simulink model "chap04_CA1"  (R2021a)
settings: Solver=FixedStepDiscrete  StartTime=0.0  StopTime=30  FixedStep=0.001  RelTol=1e-3
undefined symbols (not defined in the file): DiscIntNeverNeededParam
libraries: simulink x4
(part 2 of 4)

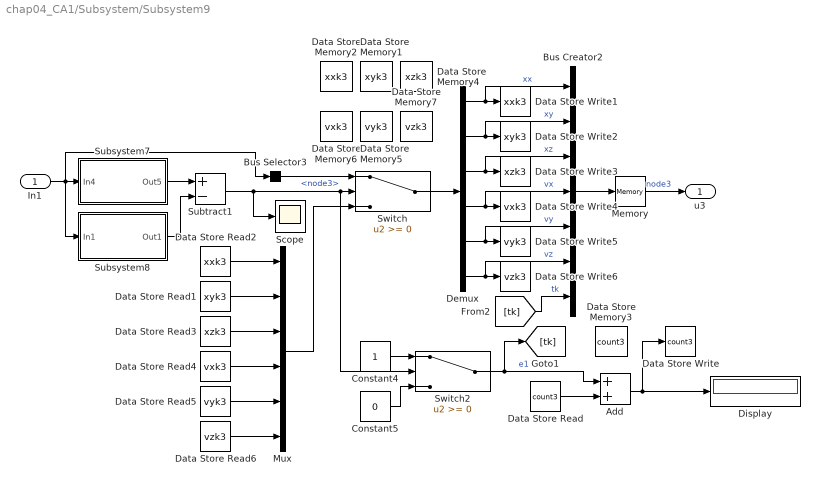
== system chap04_CA1/Subsystem/Subsystem9 ==
  In1 : Inport
  Add : Sum
  Bus Creator2 : BusCreator  Inputs=7
  Bus Selector3 : BusSelector  OutputSignals=state(t).node3
  Constant4 : Constant
  Constant5 : Constant  Value=0
  Data Store Memory1 : DataStoreMemory  DataStoreName=xyk3  ReadBeforeWriteMsg=warning  WriteAfterWriteMsg=warning  WriteAfterReadMsg=warning  ShowAdditionalParam=off
  Data Store Memory2 : DataStoreMemory  DataStoreName=xxk3  ReadBeforeWriteMsg=warning  WriteAfterWriteMsg=warning  WriteAfterReadMsg=warning  ShowAdditionalParam=off
  Data Store Memory3 : DataStoreMemory  DataStoreName=count3  ReadBeforeWriteMsg=warning  WriteAfterWriteMsg=warning  WriteAfterReadMsg=warning  ShowAdditionalParam=off
  Data Store Memory4 : DataStoreMemory  DataStoreName=xzk3  ReadBeforeWriteMsg=warning  WriteAfterWriteMsg=warning  WriteAfterReadMsg=warning  ShowAdditionalParam=off
  Data Store Memory5 : DataStoreMemory  DataStoreName=vyk3  ReadBeforeWriteMsg=warning  WriteAfterWriteMsg=warning  WriteAfterReadMsg=warning  ShowAdditionalParam=off
  Data Store Memory6 : DataStoreMemory  DataStoreName=vxk3  ReadBeforeWriteMsg=warning  WriteAfterWriteMsg=warning  WriteAfterReadMsg=warning  ShowAdditionalParam=off
  Data Store Memory7 : DataStoreMemory  DataStoreName=vzk3  ReadBeforeWriteMsg=warning  WriteAfterWriteMsg=warning  WriteAfterReadMsg=warning  ShowAdditionalParam=off
  Data Store Read : DataStoreRead  DataStoreName=count3  IndexOptions=Index vector (dialog)  Indices=1  OutputSizes=1
  Data Store Read1 : DataStoreRead  DataStoreName=xyk3  IndexOptions=Index vector (dialog)  Indices=1  OutputSizes=1
  Data Store Read2 : DataStoreRead  DataStoreName=xxk3  IndexOptions=Index vector (dialog)  Indices=1  OutputSizes=1
  Data Store Read3 : DataStoreRead  DataStoreName=xzk3  IndexOptions=Index vector (dialog)  Indices=1  OutputSizes=1
  Data Store Read4 : DataStoreRead  DataStoreName=vxk3  IndexOptions=Index vector (dialog)  Indices=1  OutputSizes=1
  Data Store Read5 : DataStoreRead  DataStoreName=vyk3  IndexOptions=Index vector (dialog)  Indices=1  OutputSizes=1
  Data Store Read6 : DataStoreRead  DataStoreName=vzk3  IndexOptions=Index vector (dialog)  Indices=1  OutputSizes=1
  Data Store Write : DataStoreWrite  DataStoreName=count3  IndexOptions=Index vector (dialog)  Indices=1  OutputSizes=1
  Data Store Write1 : DataStoreWrite  DataStoreName=xxk3  IndexOptions=Index vector (dialog)  Indices=1  OutputSizes=1
  Data Store Write2 : DataStoreWrite  DataStoreName=xyk3  IndexOptions=Index vector (dialog)  Indices=1  OutputSizes=1
  Data Store Write3 : DataStoreWrite  DataStoreName=xzk3  IndexOptions=Index vector (dialog)  Indices=1  OutputSizes=1
  Data Store Write4 : DataStoreWrite  DataStoreName=vxk3  IndexOptions=Index vector (dialog)  Indices=1  OutputSizes=1
  Data Store Write5 : DataStoreWrite  DataStoreName=vyk3  IndexOptions=Index vector (dialog)  Indices=1  OutputSizes=1
  Data Store Write6 : DataStoreWrite  DataStoreName=vzk3  IndexOptions=Index vector (dialog)  Indices=1  OutputSizes=1
  Demux : Demux  Outputs=6
  Display : Display
  Memory : Memory
  Mux : Mux  Inputs=6
  Scope : Scope
  Subsystem7 : Subsystem
  Subsystem8 : Subsystem
  Subtract1 : Sum  Inputs=+-
  Switch : Switch
  Switch2 : Switch
  u3 : Outport
  wires:
  Data Store Read6/1 -> Mux/6
  Switch/1 -> Demux/1
  Demux/2 -> Bus Creator2/2, Data Store Write2/1  "xy"
  Bus Selector3/1 -> Switch/1  "<node3>"
  Demux/1 -> Bus Creator2/1, Data Store Write1/1  "xx"
  Switch2/1 -> [tk], Add/1  "e1"
  Demux/6 -> Bus Creator2/6, Data Store Write6/1  "vz"
  Demux/3 -> Bus Creator2/3, Data Store Write3/1  "xz"
  Data Store Read2/1 -> Mux/1
  Constant4/1 -> Switch2/1
  Mux/1 -> Switch/3
  Data Store Read3/1 -> Mux/3
  Add/1 -> Data Store Write/1, Display/1
  Demux/4 -> Bus Creator2/4, Data Store Write4/1  "vx"
  Memory/1 -> u3/1  "node3"
  Data Store Read5/1 -> Mux/5
  Data Store Read4/1 -> Mux/4
  Data Store Read1/1 -> Mux/2
  Constant5/1 -> Switch2/3
  Demux/5 -> Bus Creator2/5, Data Store Write5/1  "vy"
  Data Store Read/1 -> Add/2
  Bus Creator2/1 -> Memory/1
  Subtract1/1 -> Scope/1, Switch/2, Switch2/2
  [tk] -> Bus Creator2/7  "tk"
  Subsystem8/1(Out1) -> Subtract1/2
  In1/1 -> Bus Selector3/1, Subsystem7/1(In4), Subsystem8/1(In1)
  Subsystem7/1(Out5) -> Subtract1/1

== system chap04_CA1/Subsystem2/Subsystem ==
  dx : Inport
  dy : Inport  Port=2
  dz : Inport  Port=3
  ut1x : Inport  Port=4
  ut1y : Inport  Port=5
  ut1z : Inport  Port=6
  Add : Sum
  Add1 : Sum
  Add2 : Sum
  Add3 : Sum  Inputs=-+
  Add4 : Sum  Inputs=-+
  Add5 : Sum  Inputs=-+
  Bus Creator1 : BusCreator  Inputs=6
  Constant : Constant  Value=-1
  Constant1 : Constant
  Constant2 : Constant  Value=0
  Discrete-Time Integrator{,15..17} (4 alike) : DiscreteIntegrator  SampleTime=-1  ICPrevOutput=DiscIntNeverNeededParam  ICPrevScaledInput=DiscIntNeverNeededParam
  Discrete-Time Integrator14 : DiscreteIntegrator  InitialCondition=-1  SampleTime=-1  ICPrevOutput=DiscIntNeverNeededParam  ICPrevScaledInput=DiscIntNeverNeededParam
  Discrete-Time Integrator5 : DiscreteIntegrator  InitialCondition=1  SampleTime=-1  ICPrevOutput=DiscIntNeverNeededParam  ICPrevScaledInput=DiscIntNeverNeededParam
  node1 : Outport
  wires:
  ut1y/1 -> Add1/2
  ut1z/1 -> Add2/2
  Discrete-Time Integrator17/1 -> Discrete-Time Integrator15/1, Bus Creator1/5  "vy"
  Discrete-Time Integrator/1 -> Discrete-Time Integrator5/1, Bus Creator1/6  "vz"
  ut1x/1 -> Add/2
  Discrete-Time Integrator16/1 -> Bus Creator1/4, Discrete-Time Integrator14/1  "vx"
  Bus Creator1/1 -> node1/1  "node1"
  Add5/1 -> Bus Creator1/3  "xz"
  Add4/1 -> Bus Creator1/2  "xy"
  Add3/1 -> Bus Creator1/1  "xx"
  Add/1 -> Discrete-Time Integrator16/1
  Add1/1 -> Discrete-Time Integrator17/1
  Add2/1 -> Discrete-Time Integrator/1
  dy/1 -> Add1/1
  dz/1 -> Add2/1
  dx/1 -> Add/1
  Discrete-Time Integrator14/1 -> Add3/2
  Discrete-Time Integrator5/1 -> Add5/2
  Discrete-Time Integrator15/1 -> Add4/2
  Constant/1 -> Add3/1
  Constant1/1 -> Add4/1
  Constant2/1 -> Add5/1

== system chap04_CA1/Subsystem2/Subsystem1 ==
  dx : Inport
  dy : Inport  Port=2
  dz : Inport  Port=3
  ut2x : Inport  Port=4
  ut2y : Inport  Port=5
  ut2z : Inport  Port=6
  Add : Sum
  Add1 : Sum
  Add2 : Sum
  Add3 : Sum  Inputs=-+
  Add4 : Sum  Inputs=-+
  Add5 : Sum  Inputs=-+
  Bus Creator1 : BusCreator  Inputs=6
  Constant : Constant
  Constant1 : Constant
  Constant2 : Constant  Value=0
  Discrete-Time Integrator : DiscreteIntegrator  SampleTime=-1  ICPrevOutput=DiscIntNeverNeededParam  ICPrevScaledInput=DiscIntNeverNeededParam
  Discrete-Time Integrator14 : DiscreteIntegrator  InitialCondition=1.5  SampleTime=-1  ICPrevOutput=DiscIntNeverNeededParam  ICPrevScaledInput=DiscIntNeverNeededParam
  Discrete-Time Integrator15 : DiscreteIntegrator  InitialCondition=0.5  SampleTime=-1  ICPrevOutput=DiscIntNeverNeededParam  ICPrevScaledInput=DiscIntNeverNeededParam
  Discrete-Time Integrator16 : DiscreteIntegrator  SampleTime=-1  ICPrevOutput=DiscIntNeverNeededParam  ICPrevScaledInput=DiscIntNeverNeededParam
  Discrete-Time Integrator17 : DiscreteIntegrator  SampleTime=-1  ICPrevOutput=DiscIntNeverNeededParam  ICPrevScaledInput=DiscIntNeverNeededParam
  Discrete-Time Integrator5 : DiscreteIntegrator  InitialCondition=1  SampleTime=-1  ICPrevOutput=DiscIntNeverNeededParam  ICPrevScaledInput=DiscIntNeverNeededParam
  node2 : Outport
  wires:
  Bus Creator1/1 -> node2/1  "node2"
  Discrete-Time Integrator16/1 -> Bus Creator1/4, Discrete-Time Integrator14/1  "vx"
  Discrete-Time Integrator/1 -> Discrete-Time Integrator5/1, Bus Creator1/6  "vz"
  Discrete-Time Integrator17/1 -> Bus Creator1/5, Discrete-Time Integrator15/1  "vy"
  dx/1 -> Add/1
  dy/1 -> Add1/1
  dz/1 -> Add2/1
  Add2/1 -> Discrete-Time Integrator/1
  Add1/1 -> Discrete-Time Integrator17/1
  Add/1 -> Discrete-Time Integrator16/1
  ut2x/1 -> Add/2
  ut2y/1 -> Add1/2
  ut2z/1 -> Add2/2
  Constant2/1 -> Add5/1
  Constant1/1 -> Add4/1
  Discrete-Time Integrator14/1 -> Add3/2
  Discrete-Time Integrator15/1 -> Add4/2
  Discrete-Time Integrator5/1 -> Add5/2
  Constant/1 -> Add3/1
  Add3/1 -> Bus Creator1/1  "xx"
  Add4/1 -> Bus Creator1/2  "xy"
  Add5/1 -> Bus Creator1/3  "xz"

== system chap04_CA1/Subsystem2/Subsystem2 ==
  dx : Inport
  dy : Inport  Port=2
  dz : Inport  Port=3
  ut3x : Inport  Port=4
  ut3y : Inport  Port=5
  ut3z : Inport  Port=6
  Add : Sum
  Add1 : Sum
  Add2 : Sum
  Add3 : Sum  Inputs=-+
  Add4 : Sum  Inputs=-+
  Add5 : Sum  Inputs=-+
  Bus Creator1 : BusCreator  Inputs=6
  Constant : Constant  Value=-2
  Constant1 : Constant  Value=0
  Constant2 : Constant  Value=0
  Discrete-Time Integrator : DiscreteIntegrator  SampleTime=-1  ICPrevOutput=DiscIntNeverNeededParam  ICPrevScaledInput=DiscIntNeverNeededParam
  Discrete-Time Integrator14 : DiscreteIntegrator  InitialCondition=-1  SampleTime=-1  ICPrevOutput=DiscIntNeverNeededParam  ICPrevScaledInput=DiscIntNeverNeededParam
  Discrete-Time Integrator15 : DiscreteIntegrator  InitialCondition=-1  SampleTime=-1  ICPrevOutput=DiscIntNeverNeededParam  ICPrevScaledInput=DiscIntNeverNeededParam
  Discrete-Time Integrator16 : DiscreteIntegrator  SampleTime=-1  ICPrevOutput=DiscIntNeverNeededParam  ICPrevScaledInput=DiscIntNeverNeededParam
  Discrete-Time Integrator17 : DiscreteIntegrator  SampleTime=-1  ICPrevOutput=DiscIntNeverNeededParam  ICPrevScaledInput=DiscIntNeverNeededParam
  Discrete-Time Integrator5 : DiscreteIntegrator  InitialCondition=0.5  SampleTime=-1  ICPrevOutput=DiscIntNeverNeededParam  ICPrevScaledInput=DiscIntNeverNeededParam
  node3 : Outport
  wires:
  Discrete-Time Integrator17/1 -> Discrete-Time Integrator15/1, Bus Creator1/5  "vy"
  Discrete-Time Integrator/1 -> Discrete-Time Integrator5/1, Bus Creator1/6  "vz"
  Discrete-Time Integrator16/1 -> Bus Creator1/4, Discrete-Time Integrator14/1  "vx"
  Bus Creator1/1 -> node3/1  "node3"
  ut3x/1 -> Add/2
  ut3y/1 -> Add1/2
  Add/1 -> Discrete-Time Integrator16/1
  dy/1 -> Add1/1
  Add1/1 -> Discrete-Time Integrator17/1
  Add2/1 -> Discrete-Time Integrator/1
  dz/1 -> Add2/1
  dx/1 -> Add/1
  ut3z/1 -> Add2/2
  Constant2/1 -> Add5/1
  Constant1/1 -> Add4/1
  Discrete-Time Integrator14/1 -> Add3/2
  Discrete-Time Integrator15/1 -> Add4/2
  Discrete-Time Integrator5/1 -> Add5/2
  Constant/1 -> Add3/1
  Add3/1 -> Bus Creator1/1  "xx"
  Add4/1 -> Bus Creator1/2  "xy"
  Add5/1 -> Bus Creator1/3  "xz"

== system chap04_CA1/Subsystem2/Subsystem3 ==
  dx : Inport
  dy : Inport  Port=2
  dz : Inport  Port=3
  ut4x : Inport  Port=4
  ut4y : Inport  Port=5
  ut4z : Inport  Port=6
  Add : Sum
  Add1 : Sum
  Add2 : Sum
  Add3 : Sum  Inputs=-+
  Add4 : Sum  Inputs=-+
  Add5 : Sum  Inputs=-+
  Bus Creator1 : BusCreator  Inputs=6
  Constant : Constant  Value=2
  Constant1 : Constant  Value=0
  Constant2 : Constant  Value=0
  Discrete-Time Integrator : DiscreteIntegrator  SampleTime=-1  ICPrevOutput=DiscIntNeverNeededParam  ICPrevScaledInput=DiscIntNeverNeededParam
  Discrete-Time Integrator14 : DiscreteIntegrator  InitialCondition=4  SampleTime=-1  ICPrevOutput=DiscIntNeverNeededParam  ICPrevScaledInput=DiscIntNeverNeededParam
  Discrete-Time Integrator15 : DiscreteIntegrator  InitialCondition=-1  SampleTime=-1  ICPrevOutput=DiscIntNeverNeededParam  ICPrevScaledInput=DiscIntNeverNeededParam
  Discrete-Time Integrator16 : DiscreteIntegrator  SampleTime=-1  ICPrevOutput=DiscIntNeverNeededParam  ICPrevScaledInput=DiscIntNeverNeededParam
  Discrete-Time Integrator17 : DiscreteIntegrator  SampleTime=-1  ICPrevOutput=DiscIntNeverNeededParam  ICPrevScaledInput=DiscIntNeverNeededParam
  Discrete-Time Integrator5 : DiscreteIntegrator  InitialCondition=0.5  SampleTime=-1  ICPrevOutput=DiscIntNeverNeededParam  ICPrevScaledInput=DiscIntNeverNeededParam
  node4 : Outport
  wires:
  Bus Creator1/1 -> node4/1  "node4"
  Discrete-Time Integrator16/1 -> Discrete-Time Integrator14/1, Bus Creator1/4  "vx"
  Discrete-Time Integrator/1 -> Discrete-Time Integrator5/1, Bus Creator1/6  "vz"
  Discrete-Time Integrator17/1 -> Bus Creator1/5, Discrete-Time Integrator15/1  "vy"
  ut4x/1 -> Add/2
  ut4y/1 -> Add1/2
  Add/1 -> Discrete-Time Integrator16/1
  dy/1 -> Add1/1
  Add1/1 -> Discrete-Time Integrator17/1
  Add2/1 -> Discrete-Time Integrator/1
  dz/1 -> Add2/1
  dx/1 -> Add/1
  ut4z/1 -> Add2/2
  Constant2/1 -> Add5/1
  Constant1/1 -> Add4/1
  Discrete-Time Integrator14/1 -> Add3/2
  Discrete-Time Integrator15/1 -> Add4/2
  Discrete-Time Integrator5/1 -> Add5/2
  Constant/1 -> Add3/1
  Add3/1 -> Bus Creator1/1  "xx"
  Add4/1 -> Bus Creator1/2  "xy"
  Add5/1 -> Bus Creator1/3  "xz"

== system chap04_CA1/Subsystem2/Subsystem4 ==
  dx : Inport
  dy : Inport  Port=2
  dz : Inport  Port=3
  ut5x : Inport  Port=4
  ut5y : Inport  Port=5
  ut5z : Inport  Port=6
  Add : Sum
  Add1 : Sum
  Add2 : Sum
  Add3 : Sum  Inputs=-+
  Add4 : Sum  Inputs=-+
  Add5 : Sum  Inputs=-+
  Bus Creator1 : BusCreator  Inputs=6
  Constant : Constant  Value=-1
  Constant1 : Constant  Value=-1
  Constant2 : Constant  Value=0
  Discrete-Time Integrator{,5,16..17} (4 alike) : DiscreteIntegrator  SampleTime=-1  ICPrevOutput=DiscIntNeverNeededParam  ICPrevScaledInput=DiscIntNeverNeededParam
  Discrete-Time Integrator14 : DiscreteIntegrator  InitialCondition=0.7  SampleTime=-1  ICPrevOutput=DiscIntNeverNeededParam  ICPrevScaledInput=DiscIntNeverNeededParam
  Discrete-Time Integrator15 : DiscreteIntegrator  InitialCondition=-1.7  SampleTime=-1  ICPrevOutput=DiscIntNeverNeededParam  ICPrevScaledInput=DiscIntNeverNeededParam
  node5 : Outport
  wires:
  Discrete-Time Integrator17/1 -> Discrete-Time Integrator15/1, Bus Creator1/5  "vy"
  Discrete-Time Integrator/1 -> Discrete-Time Integrator5/1, Bus Creator1/6  "vz"
  Discrete-Time Integrator16/1 -> Bus Creator1/4, Discrete-Time Integrator14/1  "vx"
  Bus Creator1/1 -> node5/1  "node5"
  ut5x/1 -> Add/2
  ut5y/1 -> Add1/2
  Add/1 -> Discrete-Time Integrator16/1
  dy/1 -> Add1/1
  Add1/1 -> Discrete-Time Integrator17/1
  Add2/1 -> Discrete-Time Integrator/1
  dz/1 -> Add2/1
  dx/1 -> Add/1
  ut5z/1 -> Add2/2
  Constant2/1 -> Add5/1
  Constant1/1 -> Add4/1
  Discrete-Time Integrator14/1 -> Add3/2
  Discrete-Time Integrator15/1 -> Add4/2
  Discrete-Time Integrator5/1 -> Add5/2
  Constant/1 -> Add3/1
  Add3/1 -> Bus Creator1/1  "xx"
  Add4/1 -> Bus Creator1/2  "xy"
  Add5/1 -> Bus Creator1/3  "xz"

== system chap04_CA1/Subsystem2/Subsystem5 ==
  dx : Inport
  dy : Inport  Port=2
  dz : Inport  Port=3
  ut6x : Inport  Port=4
  ut6y : Inport  Port=5
  ut6z : Inport  Port=6
  Add : Sum
  Add1 : Sum
  Add2 : Sum
  Add3 : Sum  Inputs=-+
  Add4 : Sum  Inputs=-+
  Add5 : Sum  Inputs=-+
  Bus Creator1 : BusCreator  Inputs=6
  Constant : Constant
  Constant1 : Constant  Value=-1
  Constant2 : Constant  Value=0
  Discrete-Time Integrator{,5,16..17} (4 alike) : DiscreteIntegrator  SampleTime=-1  ICPrevOutput=DiscIntNeverNeededParam  ICPrevScaledInput=DiscIntNeverNeededParam
  Discrete-Time Integrator14 : DiscreteIntegrator  InitialCondition=3  SampleTime=-1  ICPrevOutput=DiscIntNeverNeededParam  ICPrevScaledInput=DiscIntNeverNeededParam
  Discrete-Time Integrator15 : DiscreteIntegrator  InitialCondition=-1.5  SampleTime=-1  ICPrevOutput=DiscIntNeverNeededParam  ICPrevScaledInput=DiscIntNeverNeededParam
  node6 : Outport
  wires:
  Bus Creator1/1 -> node6/1  "node6"
  Discrete-Time Integrator16/1 -> Discrete-Time Integrator14/1, Bus Creator1/4  "vx"
  Discrete-Time Integrator/1 -> Discrete-Time Integrator5/1, Bus Creator1/6  "vz"
  Discrete-Time Integrator17/1 -> Bus Creator1/5, Discrete-Time Integrator15/1  "vy"
  ut6x/1 -> Add/2
  ut6y/1 -> Add1/2
  Add/1 -> Discrete-Time Integrator16/1
  dy/1 -> Add1/1
  Add1/1 -> Discrete-Time Integrator17/1
  Add2/1 -> Discrete-Time Integrator/1
  dz/1 -> Add2/1
  dx/1 -> Add/1
  ut6z/1 -> Add2/2
  Constant2/1 -> Add5/1
  Constant1/1 -> Add4/1
  Discrete-Time Integrator14/1 -> Add3/2
  Discrete-Time Integrator15/1 -> Add4/2
  Discrete-Time Integrator5/1 -> Add5/2
  Constant/1 -> Add3/1
  Add3/1 -> Bus Creator1/1  "xx"
  Add4/1 -> Bus Creator1/2  "xy"
  Add5/1 -> Bus Creator1/3  "xz"

== system chap04_CA1/Subsystem2/Subsystem6 ==
  Clock1 : Clock
  Constant1 : Constant  Value=0.25
  Constant3 : Constant  Value=0.25
  Constant9 : Constant  Value=0.1
  Discrete Derivative : simulink/Discrete/Discrete Derivative  gainval=1.0  ICPrevScaledInput=1000  OutMin=[]  OutMax=[]  OutDataType=fixdt(1, 16)  OutScaling=2^-10  DoSatur=off
  Discrete Derivative1 : simulink/Discrete/Discrete Derivative  gainval=1.0  ICPrevScaledInput=-0.25  OutMin=[]  OutMax=[]  OutDataType=fixdt(1, 16)  OutScaling=2^-10  DoSatur=off
  Discrete Derivative2 : simulink/Discrete/Discrete Derivative  gainval=1.0  ICPrevScaledInput=249.9  OutMin=[]  OutMax=[]  OutDataType=fixdt(1, 16)  OutScaling=2^-10  DoSatur=off
  Product{,1..3} (4 alike) : Product
  Sum : Sum  Inputs=|++
  Trigonometric Function2 : Trigonometry
  Trigonometric Function3 : Trigonometry  Operator=cos
  r : Constant
  xx : Outport
  xy : Outport  Port=2
  xz : Outport  Port=3
  vx : Outport  Port=4
  vy : Outport  Port=5
  vz : Outport  Port=6
  wires:
  Discrete Derivative/1 -> vx/1
  Discrete Derivative1/1 -> vy/1
  Sum/1 -> Discrete Derivative2/1, xz/1
  Discrete Derivative2/1 -> vz/1
  Product/1 -> xx/1, Discrete Derivative/1
  Product1/1 -> xy/1, Discrete Derivative1/1
  Product2/1 -> Trigonometric Function2/1, Trigonometric Function3/1
  Trigonometric Function3/1 -> Product/1
  Constant9/1 -> Product3/2
  Clock1/1 -> Product3/1, Product2/2
  Trigonometric Function2/1 -> Product1/2
  Constant3/1 -> Product2/1
  r/1 -> Product/2, Product1/1
  Product3/1 -> Sum/1
  Constant1/1 -> Sum/2

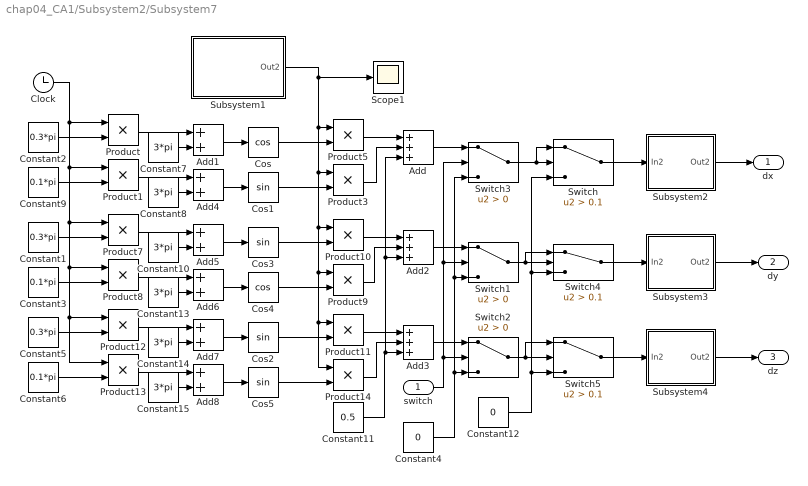
== system chap04_CA1/Subsystem2/Subsystem7 ==
  switch : Inport
  Add : Sum  Inputs=+++
  Add{1,4..8} (6 alike) : Sum
  Add2 : Sum  Inputs=+++
  Add3 : Sum  Inputs=+++
  Clock : Clock
  Constant1 : Constant  Value=0.3*pi
  Constant{7..8,10,13..15} (6 alike) : Constant  Value=3*pi
  Constant11 : Constant  Value=0.5
  Constant12 : Constant  Value=0
  Constant2 : Constant  Value=0.3*pi
  Constant3 : Constant  Value=0.1*pi
  Constant4 : Constant  Value=0
  Constant5 : Constant  Value=0.3*pi
  Constant6 : Constant  Value=0.1*pi
  Constant9 : Constant  Value=0.1*pi
  Cos : Trigonometry  Operator=cos
  Cos{1..3,5} (4 alike) : Trigonometry
  Cos4 : Trigonometry  Operator=cos
  Product{,1,3,5,7..14} (12 alike) : Product
  Scope1 : Scope
  Subsystem1 : Subsystem
  Subsystem2 : Subsystem
  Subsystem3 : Subsystem
  Subsystem4 : Subsystem
  Switch : Switch  Criteria=u2 > Threshold  Threshold=0.1
  Switch1 : Switch  Criteria=u2 > Threshold
  Switch2 : Switch  Criteria=u2 > Threshold
  Switch3 : Switch  Criteria=u2 > Threshold
  Switch4 : Switch  Criteria=u2 > Threshold  Threshold=0.1
  Switch5 : Switch  Criteria=u2 > Threshold  Threshold=0.1
  dx : Outport
  dy : Outport  Port=2
  dz : Outport  Port=3
  wires:
  Add/1 -> Switch3/1
  Add2/1 -> Switch1/1
  Switch2/1 -> Switch5/1, Switch5/2
  Product11/1 -> Add3/1
  Constant6/1 -> Product13/2
  Subsystem1/1(Out2) -> Scope1/1, Product11/1, Product14/1, Product9/1, Product10/1, Product3/1, Product5/1
  Product14/1 -> Add3/2
  Cos2/1 -> Product11/2
  Cos5/1 -> Product14/2
  Constant5/1 -> Product12/2
  Product12/1 -> Add7/1
  Product13/1 -> Add8/1
  Clock/1 -> Product/1, Product13/1, Product12/1, Product8/1, Product7/1, Product1/1
  Product10/1 -> Add2/1
  Product8/1 -> Add6/1
  Product7/1 -> Add5/1
  Constant1/1 -> Product7/2
  Cos4/1 -> Product9/2
  Cos3/1 -> Product10/2
  Product9/1 -> Add2/2
  Constant3/1 -> Product8/2
  Constant9/1 -> Product1/2
  Product3/1 -> Add/2
  Cos/1 -> Product5/2
  Add3/1 -> Switch2/1
  Cos1/1 -> Product3/2
  switch/1 -> Switch2/2, Switch1/2, Switch3/2
  Constant4/1 -> Switch3/3, Switch1/3, Switch2/3
  Product5/1 -> Add/1
  Constant2/1 -> Product/2
  Product/1 -> Add1/1
  Product1/1 -> Add4/1
  Switch1/1 -> Switch4/1, Switch4/2
  Switch3/1 -> Switch/1, Switch/2
  Switch/1 -> Subsystem2/1(In2)
  Constant12/1 -> Switch/3, Switch4/3, Switch5/3
  Constant11/1 -> Add/3, Add2/3, Add3/3
  Switch4/1 -> Subsystem3/1(In2)
  Switch5/1 -> Subsystem4/1(In2)
  Subsystem2/1(Out2) -> dx/1
  Subsystem3/1(Out2) -> dy/1
  Subsystem4/1(Out2) -> dz/1
  Add1/1 -> Cos/1
  Constant7/1 -> Add1/2
  Add4/1 -> Cos1/1
  Constant8/1 -> Add4/2
  Add5/1 -> Cos3/1
  Constant10/1 -> Add5/2
  Add6/1 -> Cos4/1
  Constant13/1 -> Add6/2
  Add7/1 -> Cos2/1
  Constant14/1 -> Add7/2
  Add8/1 -> Cos5/1
  Constant15/1 -> Add8/2

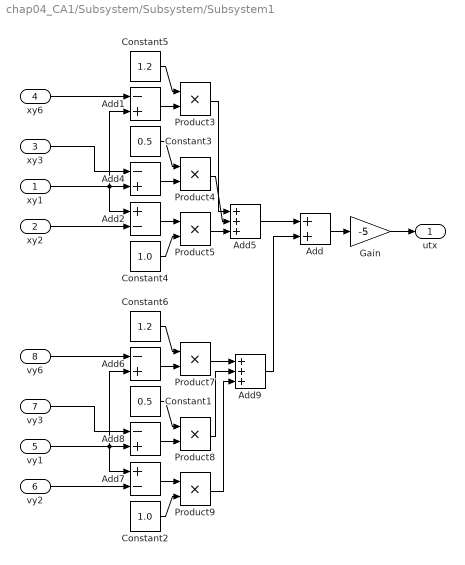
== system chap04_CA1/Subsystem/Subsystem/Subsystem1 ==
  xy1 : Inport
  xy2 : Inport  Port=2
  xy3 : Inport  Port=3
  xy6 : Inport  Port=4
  vy1 : Inport  Port=5
  vy2 : Inport  Port=6
  vy3 : Inport  Port=7
  vy6 : Inport  Port=8
  Add : Sum
  Add{1,4,6,8} (4 alike) : Sum  Inputs=-+
  Add2 : Sum  Inputs=+-
  Add5 : Sum  Inputs=+++
  Add7 : Sum  Inputs=+-
  Add9 : Sum  Inputs=+++
  Constant1 : Constant  Value=0.5
  Constant2 : Constant  Value=1.0
  Constant3 : Constant  Value=0.5
  Constant4 : Constant  Value=1.0
  Constant5 : Constant  Value=1.2
  Constant6 : Constant  Value=1.2
  Gain : Gain  Gain=-5
  Product{3..5,7..9} (6 alike) : Product
  utx : Outport
  wires:
  Product8/1 -> Add9/2
  Product9/1 -> Add9/3
  Constant1/1 -> Product8/1
  Add8/1 -> Product8/2
  vy1/1 -> Add6/2, Add8/2, Add7/1
  Constant2/1 -> Product9/2
  Add7/1 -> Product9/1
  vy3/1 -> Add8/1
  vy2/1 -> Add7/2
  vy6/1 -> Add6/1
  Constant6/1 -> Product7/1
  Add6/1 -> Product7/2
  Product7/1 -> Add9/1
  Product3/1 -> Add5/1
  Add1/1 -> Product3/2
  Constant5/1 -> Product3/1
  xy6/1 -> Add1/1
  xy2/1 -> Add2/2
  xy3/1 -> Add4/1
  Add2/1 -> Product5/1
  Constant4/1 -> Product5/2
  xy1/1 -> Add2/1, Add4/2, Add1/2
  Add4/1 -> Product4/2
  Constant3/1 -> Product4/1
  Product5/1 -> Add5/3
  Product4/1 -> Add5/2
  Add5/1 -> Add/1
  Add/1 -> Gain/1
  Gain/1 -> utx/1
  Add9/1 -> Add/2

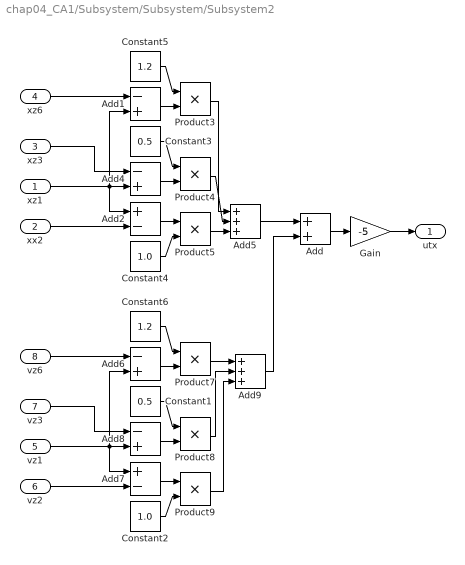
== system chap04_CA1/Subsystem/Subsystem/Subsystem2 ==
  xz1 : Inport
  xx2 : Inport  Port=2
  xz3 : Inport  Port=3
  xz6 : Inport  Port=4
  vz1 : Inport  Port=5
  vz2 : Inport  Port=6
  vz3 : Inport  Port=7
  vz6 : Inport  Port=8
  Add : Sum
  Add{1,4,6,8} (4 alike) : Sum  Inputs=-+
  Add2 : Sum  Inputs=+-
  Add5 : Sum  Inputs=+++
  Add7 : Sum  Inputs=+-
  Add9 : Sum  Inputs=+++
  Constant1 : Constant  Value=0.5
  Constant2 : Constant  Value=1.0
  Constant3 : Constant  Value=0.5
  Constant4 : Constant  Value=1.0
  Constant5 : Constant  Value=1.2
  Constant6 : Constant  Value=1.2
  Gain : Gain  Gain=-5
  Product{3..5,7..9} (6 alike) : Product
  utx : Outport
  wires:
  Product4/1 -> Add5/2
  Product5/1 -> Add5/3
  Constant3/1 -> Product4/1
  Add4/1 -> Product4/2
  xz1/1 -> Add1/2, Add4/2, Add2/1
  Constant4/1 -> Product5/2
  Add2/1 -> Product5/1
  xz3/1 -> Add4/1
  xx2/1 -> Add2/2
  xz6/1 -> Add1/1
  Constant5/1 -> Product3/1
  Add1/1 -> Product3/2
  Product3/1 -> Add5/1
  Product7/1 -> Add9/1
  Add6/1 -> Product7/2
  Constant6/1 -> Product7/1
  vz6/1 -> Add6/1
  vz2/1 -> Add7/2
  vz3/1 -> Add8/1
  Add7/1 -> Product9/1
  Constant2/1 -> Product9/2
  vz1/1 -> Add7/1, Add8/2, Add6/2
  Add8/1 -> Product8/2
  Constant1/1 -> Product8/1
  Product9/1 -> Add9/3
  Product8/1 -> Add9/2
  Add5/1 -> Add/1
  Add/1 -> Gain/1
  Gain/1 -> utx/1
  Add9/1 -> Add/2

== system chap04_CA1/Subsystem/Subsystem/Subsystem6 ==
  xx1 : Inport
  xx2 : Inport  Port=2
  xx3 : Inport  Port=3
  xx6 : Inport  Port=4
  vx1 : Inport  Port=5
  vx2 : Inport  Port=6
  vx3 : Inport  Port=7
  vx6 : Inport  Port=8
  Add : Sum
  Add{1,4,6,8} (4 alike) : Sum  Inputs=-+
  Add2 : Sum  Inputs=+-
  Add5 : Sum  Inputs=+++
  Add7 : Sum  Inputs=+-
  Add9 : Sum  Inputs=+++
  Constant1 : Constant  Value=0.5
  Constant2 : Constant  Value=1.0
  Constant3 : Constant  Value=0.5
  Constant4 : Constant  Value=1.0
  Constant5 : Constant  Value=1.2
  Constant6 : Constant  Value=1.2
  Gain : Gain  Gain=-5
  Product{3..5,7..9} (6 alike) : Product
  utx : Outport
  wires:
  Product4/1 -> Add5/2
  Product5/1 -> Add5/3
  Constant3/1 -> Product4/1
  Add4/1 -> Product4/2
  xx1/1 -> Add1/2, Add4/2, Add2/1
  Constant4/1 -> Product5/2
  Add5/1 -> Add/1
  Add9/1 -> Add/2
  Add2/1 -> Product5/1
  xx3/1 -> Add4/1
  xx2/1 -> Add2/2
  xx6/1 -> Add1/1
  Constant5/1 -> Product3/1
  Add1/1 -> Product3/2
  Product3/1 -> Add5/1
  Product7/1 -> Add9/1
  Add6/1 -> Product7/2
  Constant6/1 -> Product7/1
  vx6/1 -> Add6/1
  vx2/1 -> Add7/2
  vx3/1 -> Add8/1
  Add7/1 -> Product9/1
  Constant2/1 -> Product9/2
  vx1/1 -> Add7/1, Add8/2, Add6/2
  Add8/1 -> Product8/2
  Constant1/1 -> Product8/1
  Product9/1 -> Add9/3
  Product8/1 -> Add9/2
  Add/1 -> Gain/1
  Gain/1 -> utx/1

== system chap04_CA1/Subsystem/Subsystem1/Subsystem1 ==
  xy5 : Inport
  xy0 : Inport  Port=2
  xy3 : Inport  Port=3
  xy4 : Inport  Port=4
  vy5 : Inport  Port=5
  vy0 : Inport  Port=6
  vy3 : Inport  Port=7
  vy4 : Inport  Port=8
  Add : Sum
  Add1 : Sum  Inputs=-+
  Add10 : Sum  Inputs=-+
  Add2 : Sum  Inputs=+-
  Add4 : Sum  Inputs=-+
  Add5 : Sum  Inputs=+++
  Add6 : Sum  Inputs=+-
  Add8 : Sum  Inputs=+++
  Add9 : Sum  Inputs=+-
  Constant3 : Constant  Value=1.2
  Constant4 : Constant  Value=1.5
  Constant5 : Constant  Value=1.2
  Constant6 : Constant  Value=1.5
  Constant7 : Constant  Value=2.0
  Constant8 : Constant  Value=2.0
  Gain : Gain  Gain=-5.0
  Product{3..5,7..9} (6 alike) : Product
  uty : Outport
  wires:
  vy0/1 -> Add6/2
  Constant8/1 -> Product7/2
  Add6/1 -> Product7/1
  Product7/1 -> Add8/3
  Product3/1 -> Add5/1
  xy0/1 -> Add1/1
  Add1/1 -> Product3/2
  Constant7/1 -> Product3/1
  Product9/1 -> Add8/2
  Product8/1 -> Add8/1
  Add9/1 -> Product9/1
  Constant6/1 -> Product9/2
  Add10/1 -> Product8/2
  Constant5/1 -> Product8/1
  Product4/1 -> Add5/2
  Product5/1 -> Add5/3
  Constant3/1 -> Product4/1
  Add4/1 -> Product4/2
  xy5/1 -> Add2/1, Add4/2, Add1/2
  Constant4/1 -> Product5/2
  Add2/1 -> Product5/1
  xy4/1 -> Add4/1
  xy3/1 -> Add2/2
  vy3/1 -> Add9/2
  vy4/1 -> Add10/1
  vy5/1 -> Add9/1, Add6/1, Add10/2
  Add/1 -> Gain/1
  Gain/1 -> uty/1
  Add5/1 -> Add/1
  Add8/1 -> Add/2

== system chap04_CA1/Subsystem/Subsystem1/Subsystem2 ==
  xz5 : Inport
  xz0 : Inport  Port=2
  xz3 : Inport  Port=3
  xz4 : Inport  Port=4
  vz5 : Inport  Port=5
  vz0 : Inport  Port=6
  vz3 : Inport  Port=7
  vz4 : Inport  Port=8
  Add : Sum
  Add1 : Sum  Inputs=-+
  Add10 : Sum  Inputs=-+
  Add2 : Sum  Inputs=+-
  Add4 : Sum  Inputs=-+
  Add5 : Sum  Inputs=+++
  Add6 : Sum  Inputs=+-
  Add8 : Sum  Inputs=+++
  Add9 : Sum  Inputs=+-
  Constant3 : Constant  Value=1.2
  Constant4 : Constant  Value=1.5
  Constant5 : Constant  Value=1.2
  Constant6 : Constant  Value=1.5
  Constant7 : Constant  Value=2.0
  Constant8 : Constant  Value=2.0
  Gain : Gain  Gain=-5.0
  Product{3..5,7..9} (6 alike) : Product
  utz : Outport
  wires:
  vz5/1 -> Add10/2, Add6/1, Add9/1
  vz4/1 -> Add10/1
  vz3/1 -> Add9/2
  xz3/1 -> Add2/2
  xz4/1 -> Add4/1
  Add2/1 -> Product5/1
  Constant4/1 -> Product5/2
  xz5/1 -> Add1/2, Add4/2, Add2/1
  Add4/1 -> Product4/2
  Constant3/1 -> Product4/1
  Product5/1 -> Add5/3
  Product4/1 -> Add5/2
  Constant5/1 -> Product8/1
  Add10/1 -> Product8/2
  Constant6/1 -> Product9/2
  Add9/1 -> Product9/1
  Product8/1 -> Add8/1
  Product9/1 -> Add8/2
  Constant7/1 -> Product3/1
  Add1/1 -> Product3/2
  xz0/1 -> Add1/1
  Product3/1 -> Add5/1
  Product7/1 -> Add8/3
  Add6/1 -> Product7/1
  Constant8/1 -> Product7/2
  vz0/1 -> Add6/2
  Add/1 -> Gain/1
  Gain/1 -> utz/1
  Add5/1 -> Add/1
  Add8/1 -> Add/2

== system chap04_CA1/Subsystem/Subsystem1/Subsystem6 ==
  xx5 : Inport
  xx0 : Inport  Port=2
  xx3 : Inport  Port=3
  xx4 : Inport  Port=4
  vx5 : Inport  Port=5
  vx0 : Inport  Port=6
  vx3 : Inport  Port=7
  vx4 : Inport  Port=8
  Add : Sum
  Add1 : Sum  Inputs=-+
  Add10 : Sum  Inputs=-+
  Add2 : Sum  Inputs=+-
  Add4 : Sum  Inputs=-+
  Add5 : Sum  Inputs=+++
  Add6 : Sum  Inputs=+-
  Add8 : Sum  Inputs=+++
  Add9 : Sum  Inputs=+-
  Constant3 : Constant  Value=1.2
  Constant4 : Constant  Value=1.5
  Constant5 : Constant  Value=1.2
  Constant6 : Constant  Value=1.5
  Constant7 : Constant  Value=2.0
  Constant8 : Constant  Value=2.0
  Gain : Gain  Gain=-5.0
  Product{3..5,7..9} (6 alike) : Product
  utx : Outport
  wires:
  vx5/1 -> Add10/2, Add6/1, Add9/1
  vx4/1 -> Add10/1
  vx3/1 -> Add9/2
  xx3/1 -> Add2/2
  xx4/1 -> Add4/1
  Add2/1 -> Product5/1
  Constant4/1 -> Product5/2
  xx5/1 -> Add1/2, Add4/2, Add2/1
  Add4/1 -> Product4/2
  Constant3/1 -> Product4/1
  Product5/1 -> Add5/3
  Product4/1 -> Add5/2
  Constant5/1 -> Product8/1
  Add10/1 -> Product8/2
  Constant6/1 -> Product9/2
  Add9/1 -> Product9/1
  Product8/1 -> Add8/1
  Product9/1 -> Add8/2
  Constant7/1 -> Product3/1
  Add1/1 -> Product3/2
  xx0/1 -> Add1/1
  Product3/1 -> Add5/1
  Product7/1 -> Add8/3
  Add6/1 -> Product7/1
  Constant8/1 -> Product7/2
  vx0/1 -> Add6/2
  Add5/1 -> Add/1
  Add/1 -> Gain/1
  Gain/1 -> utx/1
  Add8/1 -> Add/2

== system chap04_CA1/Subsystem/Subsystem10/Subsystem7 ==
  In4 : Inport
  Add : Sum
  Bus Selector1 : BusSelector  OutputSignals=state(tk).node4.xx,state(t).node4.xx
  Bus Selector2 : BusSelector  OutputSignals=state(tk).node4.xy,state(t).node4.xy
  Bus Selector3 : BusSelector  OutputSignals=state(tk).node4.xz,state(t).node4.xz
  Bus Selector4 : BusSelector  OutputSignals=state(tk).node4.vx,state(t).node4.vx
  Bus Selector5 : BusSelector  OutputSignals=state(tk).node4.vy,state(t).node4.vy
  Bus Selector6 : BusSelector  OutputSignals=state(tk).node4.vz,state(t).node4.vz
  MATLAB Function1 : MATLAB Function  TreatAsAtomicUnit=on
  MATLAB Function2 : MATLAB Function  TreatAsAtomicUnit=on
  Mux1 : Mux  Inputs=3
  Mux2 : Mux  Inputs=3
  Square : Math  Operator=square  SaturateOnIntegerOverflow=on
  Square1 : Math  Operator=square  SaturateOnIntegerOverflow=on
  Subsystem3 : Subsystem
  Subsystem4 : Subsystem
  Subsystem5 : Subsystem
  Subsystem7 : Subsystem
  Subsystem8 : Subsystem
  Subsystem9 : Subsystem
  Out5 : Outport
  wires:
  Subsystem8/1(ez) -> Mux2/3
  Subsystem7/1(ey) -> Mux2/2
  Subsystem5/1(exx) -> Mux1/1
  Subsystem9/1(evx) -> Mux2/1
  Subsystem3/1(exy) -> Mux1/2
  Subsystem4/1(exz) -> Mux1/3
  Bus Selector1/1 -> Subsystem5/1(xxk)  "<xx>"
  Bus Selector3/1 -> Subsystem4/1(xzk)  "<xz>"
  Bus Selector2/2 -> Subsystem3/2(xy)  "<xy>"
  Bus Selector1/2 -> Subsystem5/2(xx)  "<xx>"
  Bus Selector2/1 -> Subsystem3/1(xyk)  "<xy>"
  Bus Selector3/2 -> Subsystem4/2(xz)  "<xz>"
  In4/1 -> Bus Selector3/1, Bus Selector2/1, Bus Selector1/1, Bus Selector4/1, Bus Selector6/1, Bus Selector5/1
  Bus Selector4/1 -> Subsystem9/1(vxk)  "<vx>"
  Bus Selector4/2 -> Subsystem9/2(vx)  "<vx>"
  Bus Selector5/1 -> Subsystem7/1(vyk)  "<vy>"
  Bus Selector5/2 -> Subsystem7/2(vy)  "<vy>"
  Bus Selector6/1 -> Subsystem8/1(vzk)  "<vz>"
  Bus Selector6/2 -> Subsystem8/2(vz)  "<vz>"
  MATLAB Function2/1(y) -> Square/1
  Mux2/1 -> MATLAB Function1/1(u)
  Square/1 -> Add/1
  Square1/1 -> Add/2
  Mux1/1 -> MATLAB Function2/1(u)
  MATLAB Function1/1(y) -> Square1/1
  Add/1 -> Out5/1

== system chap04_CA1/Subsystem/Subsystem10/Subsystem8 ==
  In1 : Inport
  Add : Sum  Inputs=+++
  Bus Selector10 : BusSelector  OutputSignals=state(tk).node4.xy,state(tk).node2.xy,state(tk).node3.xy,state(tk).node5.xy
  Bus Selector11 : BusSelector  OutputSignals=state(tk).node4.xz,state(tk).node2.xz,state(tk).node3.xz,state(tk).node5.xz
  Bus Selector6 : BusSelector  OutputSignals=state(tk).node4.vx,state(tk).node2.vx,state(tk).node3.vx,state(tk).node5.vx
  Bus Selector7 : BusSelector  OutputSignals=state(tk).node4.vy,state(tk).node2.vy,state(tk).node3.vy,state(tk).node5.vy
  Bus Selector8 : BusSelector  OutputSignals=state(tk).node4.vz,state(tk).node2.vz,state(tk).node3.vz,state(tk).node5.vz
  Bus Selector9 : BusSelector  OutputSignals=state(tk).node4.xx,state(tk).node2.xx,state(tk).node3.xx,state(tk).node5.xx
  Clock : Clock
  Constant : Constant  Value=-0.1
  Constant1 : Constant  Value=0.1
  Gain : Gain  Gain=0.1
  Gain1 : Gain  Gain=0.1
  MATLAB Function : MATLAB Function  TreatAsAtomicUnit=on
  MATLAB Function1 : MATLAB Function  TreatAsAtomicUnit=on
  Mux1 : Mux  Inputs=3
  Mux2 : Mux  Inputs=3
  Product : Product
  Product1 : Product
  Square : Math  Operator=square  SaturateOnIntegerOverflow=on
  Square1 : Math  Operator=square  SaturateOnIntegerOverflow=on
  Square2 : Math  SaturateOnIntegerOverflow=on
  Subsystem10 : Subsystem
  Subsystem11 : Subsystem
  Subsystem12 : Subsystem
  Subsystem7 : Subsystem
  Subsystem8 : Subsystem
  Subsystem9 : Subsystem
  Out1 : Outport
  wires:
  Bus Selector11/4 -> Subsystem11/4(xz5)  "<xz>"
  Bus Selector10/2 -> Subsystem10/2(xy2)  "<xy>"
  Subsystem11/1(p4z) -> Mux2/3
  Bus Selector11/1 -> Subsystem11/1(xz4)  "<xz>"
  Subsystem10/1(p4y) -> Mux2/2
  Bus Selector10/4 -> Subsystem10/4(xy5)  "<xy>"
  Bus Selector10/1 -> Subsystem10/1(xy4)  "<xy>"
  Bus Selector11/3 -> Subsystem11/3(xz3)  "<xz>"
  Subsystem12/1(p4x) -> Mux2/1
  Bus Selector10/3 -> Subsystem10/3(xy3)  "<xy>"
  Bus Selector11/2 -> Subsystem11/2(xx2)  "<xz>"
  Bus Selector7/3 -> Subsystem7/3(vy3)  "<vy>"
  Subsystem9/1(p4x) -> Mux1/1
  Bus Selector6/2 -> Subsystem9/2(vx2)  "<vx>"
  Bus Selector7/2 -> Subsystem7/2(vy2)  "<vy>"
  Bus Selector8/2 -> Subsystem8/2(vz2)  "<vz>"
  Bus Selector6/1 -> Subsystem9/1(vx4)  "<vx>"
  Bus Selector6/3 -> Subsystem9/3(vx3)  "<vx>"
  Bus Selector7/1 -> Subsystem7/1(vy4)  "<vy>"
  Bus Selector8/4 -> Subsystem8/4(vz5)  "<vz>"
  Bus Selector7/4 -> Subsystem7/4(vy5)  "<vy>"
  In1/1 -> Bus Selector6/1, Bus Selector8/1, Bus Selector7/1, Bus Selector11/1, Bus Selector10/1, Bus Selector9/1
  Bus Selector6/4 -> Subsystem9/4(vx5)  "<vx>"
  Bus Selector8/3 -> Subsystem8/3(vz3)  "<vz>"
  Bus Selector8/1 -> Subsystem8/1(vz4)  "<vz>"
  Subsystem7/1(p4y) -> Mux1/2
  Subsystem8/1(p4z) -> Mux1/3
  Bus Selector9/1 -> Subsystem12/1(xx4)  "<xx>"
  Bus Selector9/2 -> Subsystem12/2(xx2)  "<xx>"
  Bus Selector9/3 -> Subsystem12/3(xx3)  "<xx>"
  Bus Selector9/4 -> Subsystem12/4(xx5)  "<xx>"
  Product/1 -> Add/2
  MATLAB Function/1(y) -> Square/1
  MATLAB Function1/1(y) -> Square1/1
  Square/1 -> Gain1/1
  Gain1/1 -> Add/1
  Square2/1 -> Product/1
  Constant/1 -> Product1/2
  Product1/1 -> Square2/1
  Square1/1 -> Gain/1
  Constant1/1 -> Product/2
  Clock/1 -> Product1/1
  Gain/1 -> Add/3
  Mux2/1 -> MATLAB Function/1(u)
  Add/1 -> Out1/1
  Mux1/1 -> MATLAB Function1/1(u)

== system chap04_CA1/Subsystem/Subsystem11/Subsystem7 ==
  In4 : Inport
  Add : Sum
  Bus Selector1 : BusSelector  OutputSignals=state(tk).node6.xx,state(t).node6.xx
  Bus Selector2 : BusSelector  OutputSignals=state(tk).node6.xy,state(t).node6.xy
  Bus Selector3 : BusSelector  OutputSignals=state(tk).node6.xz,state(t).node6.xz
  Bus Selector4 : BusSelector  OutputSignals=state(tk).node6.vx,state(t).node6.vx
  Bus Selector5 : BusSelector  OutputSignals=state(tk).node6.vy,state(t).node6.vy
  Bus Selector6 : BusSelector  OutputSignals=state(tk).node6.vz,state(t).node6.vz
  MATLAB Function1 : MATLAB Function  TreatAsAtomicUnit=on
  MATLAB Function2 : MATLAB Function  TreatAsAtomicUnit=on
  Mux1 : Mux  Inputs=3
  Mux2 : Mux  Inputs=3
  Square : Math  Operator=square  SaturateOnIntegerOverflow=on
  Square1 : Math  Operator=square  SaturateOnIntegerOverflow=on
  Subsystem3 : Subsystem
  Subsystem4 : Subsystem
  Subsystem5 : Subsystem
  Subsystem7 : Subsystem
  Subsystem8 : Subsystem
  Subsystem9 : Subsystem
  Out5 : Outport
  wires:
  Subsystem8/1(ez) -> Mux2/3
  Subsystem7/1(ey) -> Mux2/2
  Subsystem5/1(exx) -> Mux1/1
  Subsystem9/1(evx) -> Mux2/1
  Subsystem3/1(exy) -> Mux1/2
  Subsystem4/1(exz) -> Mux1/3
  Bus Selector1/1 -> Subsystem5/1(xxk)  "<xx>"
  Bus Selector3/1 -> Subsystem4/1(xzk)  "<xz>"
  Bus Selector2/2 -> Subsystem3/2(xy)  "<xy>"
  Bus Selector1/2 -> Subsystem5/2(xx)  "<xx>"
  Bus Selector2/1 -> Subsystem3/1(xyk)  "<xy>"
  Bus Selector3/2 -> Subsystem4/2(xz)  "<xz>"
  In4/1 -> Bus Selector3/1, Bus Selector2/1, Bus Selector1/1, Bus Selector4/1, Bus Selector6/1, Bus Selector5/1
  Bus Selector4/1 -> Subsystem9/1(vxk)  "<vx>"
  Bus Selector4/2 -> Subsystem9/2(vx)  "<vx>"
  Bus Selector5/1 -> Subsystem7/1(vyk)  "<vy>"
  Bus Selector5/2 -> Subsystem7/2(vy)  "<vy>"
  Bus Selector6/1 -> Subsystem8/1(vzk)  "<vz>"
  Bus Selector6/2 -> Subsystem8/2(vz)  "<vz>"
  MATLAB Function2/1(y) -> Square/1
  Mux2/1 -> MATLAB Function1/1(u)
  Square/1 -> Add/1
  Square1/1 -> Add/2
  Mux1/1 -> MATLAB Function2/1(u)
  MATLAB Function1/1(y) -> Square1/1
  Add/1 -> Out5/1

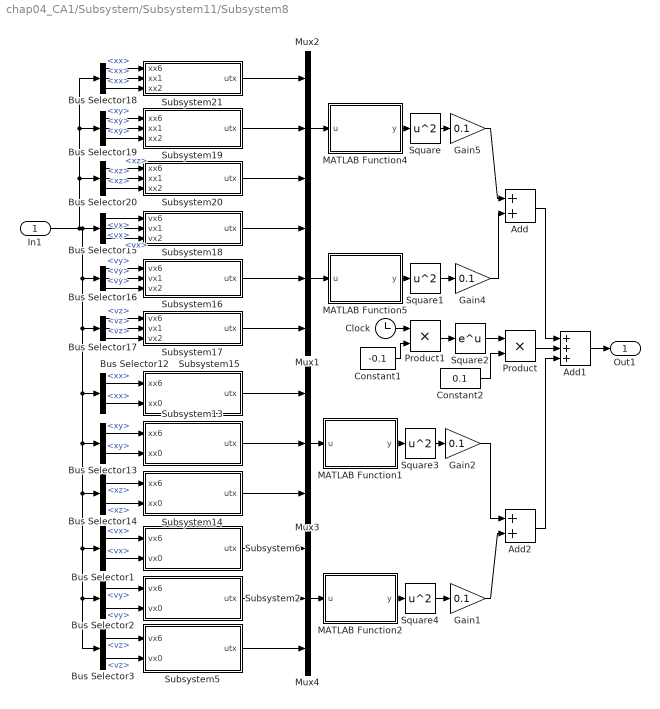
== system chap04_CA1/Subsystem/Subsystem11/Subsystem8 ==
  In1 : Inport
  Add : Sum
  Add1 : Sum  Inputs=+++
  Add2 : Sum
  Bus Selector1 : BusSelector  OutputSignals=state(t).node6.vx,state(t).node0.vx
  Bus Selector12 : BusSelector  OutputSignals=state(t).node6.xx,state(t).node0.xx
  Bus Selector13 : BusSelector  OutputSignals=state(t).node6.xy,state(t).node0.xy
  Bus Selector14 : BusSelector  OutputSignals=state(t).node6.xz,state(t).node0.xz
  Bus Selector15 : BusSelector  OutputSignals=state(tk).node6.vx,state(tk).node1.vx,state(tk).node2.vx
  Bus Selector16 : BusSelector  OutputSignals=state(tk).node6.vy,state(tk).node1.vy,state(tk).node2.vy
  Bus Selector17 : BusSelector  OutputSignals=state(tk).node6.vz,state(tk).node1.vz,state(tk).node2.vz
  Bus Selector18 : BusSelector  OutputSignals=state(tk).node6.xx,state(tk).node1.xx,state(tk).node2.xx
  Bus Selector19 : BusSelector  OutputSignals=state(tk).node6.xy,state(tk).node1.xy,state(tk).node2.xy
  Bus Selector2 : BusSelector  OutputSignals=state(t).node6.vy,state(t).node0.vy
  Bus Selector20 : BusSelector  OutputSignals=state(tk).node6.xz,state(tk).node1.xz,state(tk).node2.xz
  Bus Selector3 : BusSelector  OutputSignals=state(t).node6.vz,state(t).node0.vz
  Clock : Clock
  Constant1 : Constant  Value=-0.1
  Constant2 : Constant  Value=0.1
  Gain{1..2,4..5} (4 alike) : Gain  Gain=0.1
  MATLAB Function1 : MATLAB Function  TreatAsAtomicUnit=on
  MATLAB Function2 : MATLAB Function  TreatAsAtomicUnit=on
  MATLAB Function4 : MATLAB Function  TreatAsAtomicUnit=on
  MATLAB Function5 : MATLAB Function  TreatAsAtomicUnit=on
  Mux{1..4} (4 alike) : Mux  Inputs=3
  Product : Product
  Product1 : Product
  Square{,1,3..4} (4 alike) : Math  Operator=square  SaturateOnIntegerOverflow=on
  Square2 : Math  SaturateOnIntegerOverflow=on
  Subsystem13 : Subsystem
  Subsystem14 : Subsystem
  Subsystem15 : Subsystem
  Subsystem16 : Subsystem
  Subsystem17 : Subsystem
  Subsystem18 : Subsystem
  Subsystem19 : Subsystem
  Subsystem2 : Subsystem
  Subsystem20 : Subsystem
  Subsystem21 : Subsystem
  Subsystem5 : Subsystem
  Subsystem6 : Subsystem
  Out1 : Outport
  wires:
  Subsystem20/1(utx) -> Mux2/3
  Subsystem19/1(utx) -> Mux2/2
  Subsystem21/1(utx) -> Mux2/1
  Subsystem18/1(utx) -> Mux1/1
  In1/1 -> Bus Selector19/1, Bus Selector18/1, Bus Selector20/1, Bus Selector15/1, Bus Selector17/1, Bus Selector12/1, Bus Selector13/1, Bus Selector1/1, Bus Selector3/1, Bus Selector2/1, Bus Selector14/1, Bus Selector16/1
  Subsystem16/1(utx) -> Mux1/2
  Subsystem17/1(utx) -> Mux1/3
  Bus Selector16/2 -> Subsystem16/2(vx1)  "<vy>"
  Bus Selector16/1 -> Subsystem16/1(vx6)  "<vy>"
  Bus Selector16/3 -> Subsystem16/3(vx2)  "<vy>"
  Bus Selector15/1 -> Subsystem18/1(vx6)  "<vx>"
  Bus Selector15/2 -> Subsystem18/2(vx1)  "<vx>"
  Bus Selector15/3 -> Subsystem18/3(vx2)  "<vx>"
  Bus Selector17/3 -> Subsystem17/3(vx2)  "<vz>"
  Bus Selector17/2 -> Subsystem17/2(vx1)  "<vz>"
  Bus Selector17/1 -> Subsystem17/1(vx6)  "<vz>"
  Subsystem14/1(utx) -> Mux3/3
  Subsystem13/1(utx) -> Mux3/2
  Subsystem15/1(utx) -> Mux3/1
  Subsystem6/1(utx) -> Mux4/1
  Subsystem2/1(utx) -> Mux4/2
  Subsystem5/1(utx) -> Mux4/3
  Bus Selector12/2 -> Subsystem15/2(xx0)  "<xx>"
  Bus Selector12/1 -> Subsystem15/1(xx6)  "<xx>"
  Bus Selector14/1 -> Subsystem14/1(xx6)  "<xz>"
  Bus Selector14/2 -> Subsystem14/2(xx0)  "<xz>"
  Bus Selector1/1 -> Subsystem6/1(vx6)  "<vx>"
  Bus Selector1/2 -> Subsystem6/2(vx0)  "<vx>"
  Bus Selector2/1 -> Subsystem2/1(vx6)  "<vy>"
  Bus Selector2/2 -> Subsystem2/2(vx0)  "<vy>"
  Bus Selector3/1 -> Subsystem5/1(vx6)  "<vz>"
  Bus Selector3/2 -> Subsystem5/2(vx0)  "<vz>"
  Bus Selector20/2 -> Subsystem20/2(xx1)  "<xz>"
  Bus Selector18/2 -> Subsystem21/2(xx1)  "<xx>"
  Bus Selector18/1 -> Subsystem21/1(xx6)  "<xx>"
  Bus Selector19/2 -> Subsystem19/2(xx1)  "<xy>"
  Bus Selector19/1 -> Subsystem19/1(xx6)  "<xy>"
  Bus Selector20/1 -> Subsystem20/1(xx6)  "<xz>"
  Bus Selector20/3 -> Subsystem20/3(xx2)  "<xz>"
  Bus Selector19/3 -> Subsystem19/3(xx2)  "<xy>"
  Bus Selector18/3 -> Subsystem21/3(xx2)  "<xx>"
  Mux4/1 -> MATLAB Function2/1(u)
  Clock/1 -> Product1/1
  Mux2/1 -> MATLAB Function4/1(u)
  MATLAB Function5/1(y) -> Square1/1
  Product1/1 -> Square2/1
  Square1/1 -> Gain4/1
  Square2/1 -> Product/1
  Constant2/1 -> Product/2
  MATLAB Function4/1(y) -> Square/1
  Square/1 -> Gain5/1
  Product/1 -> Add1/2
  Mux3/1 -> MATLAB Function1/1(u)
  Gain2/1 -> Add2/1
  Mux1/1 -> MATLAB Function5/1(u)
  Gain1/1 -> Add2/2
  Gain4/1 -> Add/2
  MATLAB Function2/1(y) -> Square4/1
  MATLAB Function1/1(y) -> Square3/1
  Square4/1 -> Gain1/1
  Square3/1 -> Gain2/1
  Add2/1 -> Add1/3
  Gain5/1 -> Add/1
  Add/1 -> Add1/1
  Constant1/1 -> Product1/2
  Add1/1 -> Out1/1
  Bus Selector13/1 -> Subsystem13/1(xx6)  "<xy>"
  Bus Selector13/2 -> Subsystem13/2(xx0)  "<xy>"

== system chap04_CA1/Subsystem/Subsystem13/Subsystem3 ==
  In4 : Inport
  Add : Sum
  Bus Selector1 : BusSelector  OutputSignals=state(tk).node2.vx,state(t).node2.vx
  Bus Selector2 : BusSelector  OutputSignals=state(tk).node2.vy,state(t).node2.vy
  Bus Selector3 : BusSelector  OutputSignals=state(tk).node2.vz,state(t).node2.vz
  Bus Selector4 : BusSelector  OutputSignals=state(tk).node2.xx,state(t).node2.xx
  Bus Selector5 : BusSelector  OutputSignals=state(tk).node2.xy,state(t).node2.xy
  Bus Selector6 : BusSelector  OutputSignals=state(tk).node2.xz,state(t).node2.xz
  MATLAB Function1 : MATLAB Function  TreatAsAtomicUnit=on
  MATLAB Function2 : MATLAB Function  TreatAsAtomicUnit=on
  Mux1 : Mux  Inputs=3
  Mux2 : Mux  Inputs=3
  Square : Math  Operator=square  SaturateOnIntegerOverflow=on
  Square1 : Math  Operator=square  SaturateOnIntegerOverflow=on
  Subsystem3 : Subsystem
  Subsystem4 : Subsystem
  Subsystem5 : Subsystem
  Subsystem7 : Subsystem
  Subsystem8 : Subsystem
  Subsystem9 : Subsystem
  Out5 : Outport
  wires:
  Subsystem8/1(ez) -> Mux2/3
  Subsystem7/1(ey) -> Mux2/2
  Subsystem5/1(exx) -> Mux1/1
  Subsystem9/1(evx) -> Mux2/1
  Subsystem3/1(exy) -> Mux1/2
  Subsystem4/1(exz) -> Mux1/3
  Mux1/1 -> MATLAB Function2/1(u)
  Add/1 -> Out5/1
  Mux2/1 -> MATLAB Function1/1(u)
  MATLAB Function1/1(y) -> Square1/1
  MATLAB Function2/1(y) -> Square/1
  Square/1 -> Add/1
  Square1/1 -> Add/2
  Bus Selector4/1 -> Subsystem5/1(xxk)  "<xx>"
  Bus Selector6/1 -> Subsystem4/1(xzk)  "<xz>"
  Bus Selector5/2 -> Subsystem3/2(xy)  "<xy>"
  Bus Selector4/2 -> Subsystem5/2(xx)  "<xx>"
  Bus Selector5/1 -> Subsystem3/1(xyk)  "<xy>"
  Bus Selector6/2 -> Subsystem4/2(xz)  "<xz>"
  In4/1 -> Bus Selector4/1, Bus Selector5/1, Bus Selector2/1, Bus Selector3/1, Bus Selector1/1, Bus Selector6/1
  Bus Selector1/1 -> Subsystem9/1(vxk)  "<vx>"
  Bus Selector1/2 -> Subsystem9/2(vx)  "<vx>"
  Bus Selector2/1 -> Subsystem7/1(vyk)  "<vy>"
  Bus Selector2/2 -> Subsystem7/2(vy)  "<vy>"
  Bus Selector3/1 -> Subsystem8/1(vzk)  "<vz>"
  Bus Selector3/2 -> Subsystem8/2(vz)  "<vz>"

== system chap04_CA1/Subsystem/Subsystem13/Subsystem7 ==
  In1 : Inport
  Add : Sum  Inputs=+++
  Bus Selector10 : BusSelector  OutputSignals=state(tk).node2.xy,state(tk).node1.xy,state(tk).node4.xy,state(tk).node6.xy
  Bus Selector11 : BusSelector  OutputSignals=state(tk).node2.xz,state(tk).node1.xz,state(tk).node4.xz,state(tk).node6.xz
  Bus Selector6 : BusSelector  OutputSignals=state(tk).node2.vx,state(tk).node1.vx,state(tk).node4.vx,state(tk).node6.vx
  Bus Selector7 : BusSelector  OutputSignals=state(tk).node2.vy,state(tk).node1.vy,state(tk).node4.vy,state(tk).node6.vy
  Bus Selector8 : BusSelector  OutputSignals=state(tk).node2.vz,state(tk).node1.vz,state(tk).node4.vz,state(tk).node6.vz
  Bus Selector9 : BusSelector  OutputSignals=state(tk).node2.xx,state(tk).node1.xx,state(tk).node4.xx,state(tk).node6.xx
  Clock : Clock
  Constant : Constant  Value=-0.1
  Constant1 : Constant  Value=0.1
  Gain : Gain  Gain=0.1
  Gain1 : Gain  Gain=0.1
  MATLAB Function : MATLAB Function  TreatAsAtomicUnit=on
  MATLAB Function1 : MATLAB Function  TreatAsAtomicUnit=on
  Mux1 : Mux  Inputs=3
  Mux2 : Mux  Inputs=3
  Product : Product
  Product1 : Product
  Square : Math  Operator=square  SaturateOnIntegerOverflow=on
  Square1 : Math  Operator=square  SaturateOnIntegerOverflow=on
  Square2 : Math  SaturateOnIntegerOverflow=on
  Subsystem10 : Subsystem
  Subsystem11 : Subsystem
  Subsystem12 : Subsystem
  Subsystem7 : Subsystem
  Subsystem8 : Subsystem
  Subsystem9 : Subsystem
  Out1 : Outport
  wires:
  Bus Selector11/4 -> Subsystem11/4(xz6)  "<xz>"
  Bus Selector10/2 -> Subsystem10/2(xy1)  "<xy>"
  Subsystem11/1(p2z) -> Mux2/3
  Bus Selector11/1 -> Subsystem11/1(xz2)  "<xz>"
  Subsystem10/1(p2y) -> Mux2/2
  Bus Selector10/4 -> Subsystem10/4(xy6)  "<xy>"
  Bus Selector10/1 -> Subsystem10/1(xy2)  "<xy>"
  Bus Selector11/3 -> Subsystem11/3(xz4)  "<xz>"
  Subsystem12/1(p2x) -> Mux2/1
  Bus Selector10/3 -> Subsystem10/3(xy4)  "<xy>"
  Bus Selector11/2 -> Subsystem11/2(xz1)  "<xz>"
  Bus Selector7/3 -> Subsystem7/3(vy4)  "<vy>"
  Subsystem9/1(p2x) -> Mux1/1
  Bus Selector6/2 -> Subsystem9/2(vx1)  "<vx>"
  Bus Selector7/2 -> Subsystem7/2(vy1)  "<vy>"
  Bus Selector8/2 -> Subsystem8/2(vz1)  "<vz>"
  Bus Selector6/1 -> Subsystem9/1(vx2)  "<vx>"
  Bus Selector6/3 -> Subsystem9/3(vx4)  "<vx>"
  Bus Selector7/1 -> Subsystem7/1(vy2)  "<vy>"
  Bus Selector8/4 -> Subsystem8/4(vz6)  "<vz>"
  Bus Selector7/4 -> Subsystem7/4(vy6)  "<vy>"
  In1/1 -> Bus Selector8/1, Bus Selector7/1, Bus Selector6/1, Bus Selector9/1, Bus Selector10/1, Bus Selector11/1
  Bus Selector6/4 -> Subsystem9/4(vx6)  "<vx>"
  Bus Selector8/3 -> Subsystem8/3(vz4)  "<vz>"
  Bus Selector8/1 -> Subsystem8/1(vz2)  "<vz>"
  Subsystem7/1(p2y) -> Mux1/2
  Subsystem8/1(p2z) -> Mux1/3
  Bus Selector9/1 -> Subsystem12/1(xx2)  "<xx>"
  Bus Selector9/2 -> Subsystem12/2(xx1)  "<xx>"
  Bus Selector9/3 -> Subsystem12/3(xx4)  "<xx>"
  Bus Selector9/4 -> Subsystem12/4(xx6)  "<xx>"
  Constant/1 -> Product1/2
  Square2/1 -> Product/1
  Constant1/1 -> Product/2
  Square1/1 -> Gain/1
  Gain/1 -> Add/3
  Product1/1 -> Square2/1
  Clock/1 -> Product1/1
  Add/1 -> Out1/1
  MATLAB Function/1(y) -> Square/1
  Mux1/1 -> MATLAB Function1/1(u)
  Square/1 -> Gain1/1
  MATLAB Function1/1(y) -> Square1/1
  Gain1/1 -> Add/1
  Mux2/1 -> MATLAB Function/1(u)
  Product/1 -> Add/2

== system chap04_CA1/Subsystem/Subsystem2/Subsystem1 ==
  xy2 : Inport
  xy1 : Inport  Port=2
  xy4 : Inport  Port=3
  xy6 : Inport  Port=4
  vy2 : Inport  Port=5
  vy1 : Inport  Port=6
  vy4 : Inport  Port=7
  vy6 : Inport  Port=8
  Add : Sum
  Add{1,4,6,8} (4 alike) : Sum  Inputs=-+
  Add2 : Sum  Inputs=+-
  Add5 : Sum  Inputs=+++
  Add7 : Sum  Inputs=+-
  Add9 : Sum  Inputs=+++
  Constant1 : Constant  Value=0.5
  Constant2 : Constant  Value=1.0
  Constant3 : Constant  Value=0.5
  Constant4 : Constant  Value=1.0
  Constant5 : Constant  Value=1.5
  Constant6 : Constant  Value=1.5
  Gain : Gain  Gain=-5
  Product{3..5,7..9} (6 alike) : Product
  p2y : Outport
  wires:
  Product8/1 -> Add9/2
  Product9/1 -> Add9/3
  Constant1/1 -> Product8/1
  Add8/1 -> Product8/2
  vy2/1 -> Add6/2, Add8/2, Add7/1
  Constant2/1 -> Product9/2
  Add7/1 -> Product9/1
  vy4/1 -> Add8/1
  vy1/1 -> Add7/2
  vy6/1 -> Add6/1
  Constant6/1 -> Product7/1
  Add6/1 -> Product7/2
  Product7/1 -> Add9/1
  Product3/1 -> Add5/1
  Add1/1 -> Product3/2
  Constant5/1 -> Product3/1
  xy6/1 -> Add1/1
  xy1/1 -> Add2/2
  xy4/1 -> Add4/1
  Add2/1 -> Product5/1
  Constant4/1 -> Product5/2
  xy2/1 -> Add2/1, Add4/2, Add1/2
  Add4/1 -> Product4/2
  Constant3/1 -> Product4/1
  Product5/1 -> Add5/3
  Product4/1 -> Add5/2
  Add5/1 -> Add/1
  Add/1 -> Gain/1
  Gain/1 -> p2y/1
  Add9/1 -> Add/2

== system chap04_CA1/Subsystem/Subsystem2/Subsystem2 ==
  xz2 : Inport
  xz1 : Inport  Port=2
  xz4 : Inport  Port=3
  xz6 : Inport  Port=4
  vz2 : Inport  Port=5
  vz1 : Inport  Port=6
  vz4 : Inport  Port=7
  vz6 : Inport  Port=8
  Add : Sum
  Add{1,4,6,8} (4 alike) : Sum  Inputs=-+
  Add2 : Sum  Inputs=+-
  Add5 : Sum  Inputs=+++
  Add7 : Sum  Inputs=+-
  Add9 : Sum  Inputs=+++
  Constant1 : Constant  Value=0.5
  Constant2 : Constant  Value=1.0
  Constant3 : Constant  Value=0.5
  Constant4 : Constant  Value=1.0
  Constant5 : Constant  Value=1.5
  Constant6 : Constant  Value=1.5
  Gain : Gain  Gain=-5
  Product{3..5,7..9} (6 alike) : Product
  p2z : Outport
  wires:
  Product4/1 -> Add5/2
  Product5/1 -> Add5/3
  Constant3/1 -> Product4/1
  Add4/1 -> Product4/2
  xz2/1 -> Add1/2, Add4/2, Add2/1
  Constant4/1 -> Product5/2
  Add2/1 -> Product5/1
  xz4/1 -> Add4/1
  xz1/1 -> Add2/2
  xz6/1 -> Add1/1
  Constant5/1 -> Product3/1
  Add1/1 -> Product3/2
  Product3/1 -> Add5/1
  Product7/1 -> Add9/1
  Add6/1 -> Product7/2
  Constant6/1 -> Product7/1
  vz6/1 -> Add6/1
  vz1/1 -> Add7/2
  vz4/1 -> Add8/1
  Add7/1 -> Product9/1
  Constant2/1 -> Product9/2
  vz2/1 -> Add7/1, Add8/2, Add6/2
  Add8/1 -> Product8/2
  Constant1/1 -> Product8/1
  Product9/1 -> Add9/3
  Product8/1 -> Add9/2
  Add5/1 -> Add/1
  Add/1 -> Gain/1
  Gain/1 -> p2z/1
  Add9/1 -> Add/2
